simulink model "test01_Accumulator"  (Simulink 7.4)
settings: Solver=ode45  StartTime=0.0  StopTime=1.0  RelTol=1e-3
libraries: NAV420Lib x1
settings Model: Creator=djulzz  LastModifiedBy=djulzz

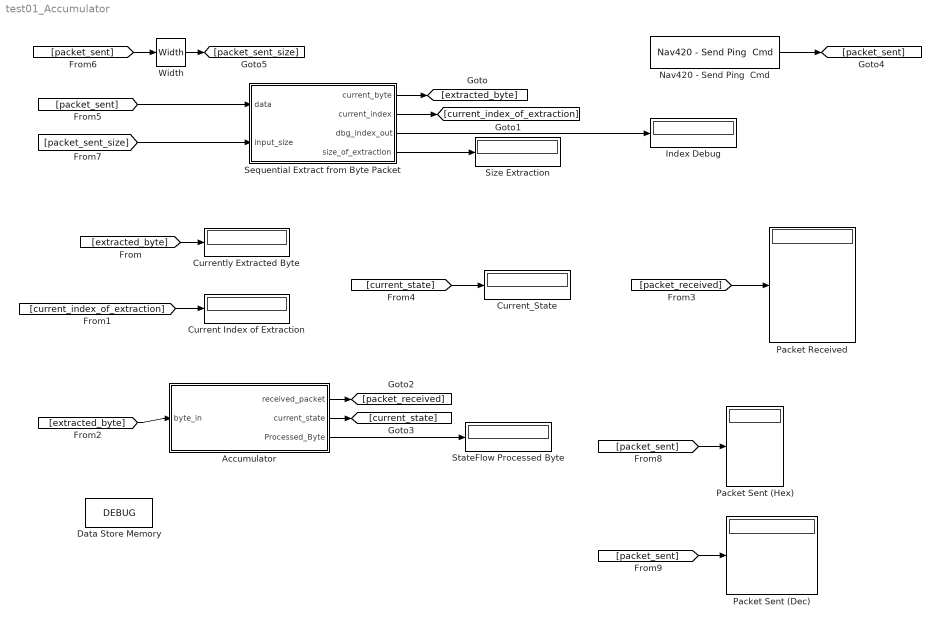
== system test01_Accumulator ==
  Accumulator : Subsystem
  Current Index of Extraction : Display
  Current_State : Display
  Currently Extracted Byte : Display
  Data Store Memory : DataStoreMemory  DataStoreName=DEBUG  DataType=double  OutDataType=fixdt(1, 16)  OutScaling=2^0  OutDataTypeStr=double
  Index Debug : Display
  Nav420 - Send Ping  Cmd : NAV420Lib/Nav420 - Send Ping  Cmd  SystemSampleTime=-1
  Packet Received : Display
  Packet Sent (Dec) : Display
  Packet Sent (Hex) : Display
      settings: Format=hex (Stored Integer)
  Sequential Extract from Byte Packet : Subsystem  TreatAsAtomicUnit=on
  Size Extraction : Display
  StateFlow Processed Byte : Display
      settings: Format=hex (Stored Integer)
  Width : Width
  wires:
  [extracted_byte] -> Currently Extracted Byte/1
  Sequential Extract from Byte Packet/1(current_byte) -> [extracted_byte]
  Sequential Extract from Byte Packet/2(current_index) -> [current_index_of_extraction]
  [current_index_of_extraction] -> Current Index of Extraction/1
  [extracted_byte] -> Accumulator/1(byte_in)
  Accumulator/1(received_packet) -> [packet_received]
  [packet_received] -> Packet Received/1
  [current_state] -> Current_State/1
  Accumulator/2(current_state) -> [current_state]
  Nav420 - Send Ping  Cmd/1 -> [packet_sent]
  [packet_sent] -> Sequential Extract from Byte Packet/1(data)
  [packet_sent] -> Width/1
  Width/1 -> [packet_sent_size]
  [packet_sent_size] -> Sequential Extract from Byte Packet/2(input_size)
  [packet_sent] -> Packet Sent (Hex)/1
  [packet_sent] -> Packet Sent (Dec)/1
  Accumulator/3(Processed_Byte) -> StateFlow Processed Byte/1
  Sequential Extract from Byte Packet/3(dbg_index_out) -> Index Debug/1
  Sequential Extract from Byte Packet/4(size_of_extraction) -> Size Extraction/1

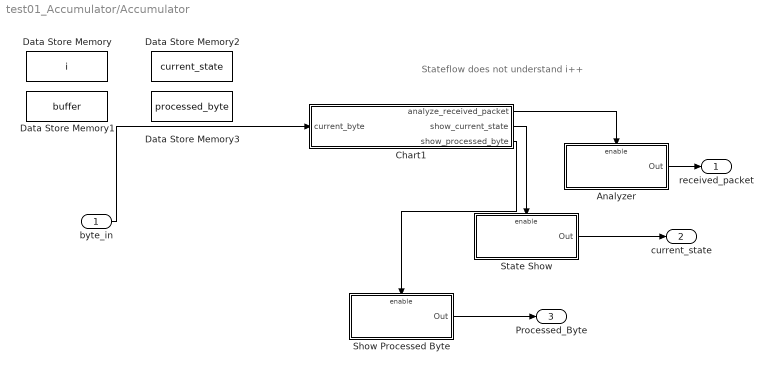
== system test01_Accumulator/Accumulator ==
  note: Stateflow does not understand i++
  byte_in : Inport  OutMin=[0]  OutMax=[255]  DataType=uint8  OutDataType=fixdt(1, 16)  OutScaling=2^0  OutDataTypeStr=uint8
  Analyzer : Subsystem  TreatAsAtomicUnit=on
  Chart1 : Stateflow chart
  Data Store Memory : DataStoreMemory  DataStoreName=i  InitialValue=1  OutMin=[0]  OutMax=[255]  DataType=uint8  OutDataType=fixdt(1, 16)  OutScaling=2^0  OutDataTypeStr=uint8
  Data Store Memory1 : DataStoreMemory  DataStoreName=buffer  InitialValue=[0 0 0 0 0 0 0 0 0 0 0 0 0 0 0 0 0 0 0 0 0 0 0 0 0 0 0 0 0 0 0 0 0 0 0 0 0 0 0 0 0 0 0 0 0 0 0 0 0 0 0 0 0 0 0 0 0 0 0 0 0 0 0 0 0 0 0 0 0 0 0 0 0 0 0 0 0 0 0 0 0 0 0 0 0 0 0 0 0 0 0 0 0 0 0 0 0 0 0 0]  DataType=uint8  OutDataType=fixdt(1, 16)  OutScaling=2^0  OutDataTypeStr=uint8
  Data Store Memory2 : DataStoreMemory  DataStoreName=current_state  DataType=double  OutDataType=fixdt(1, 16)  OutScaling=2^0  OutDataTypeStr=double
  Data Store Memory3 : DataStoreMemory  DataStoreName=processed_byte  DataType=uint8  OutDataType=fixdt(1, 16)  OutScaling=2^0  OutDataTypeStr=uint8
  Show Processed Byte : Subsystem  TreatAsAtomicUnit=on
  State Show : Subsystem  TreatAsAtomicUnit=on
  received_packet : Outport  DataType=uint8  OutDataType=fixdt(1, 16)  OutScaling=2^0  OutDataTypeStr=uint8
  current_state : Outport  Port=2  DataType=double  OutDataType=fixdt(1, 16)  OutScaling=2^0  OutDataTypeStr=double
  Processed_Byte : Outport  Port=3  DataType=uint8  OutDataType=fixdt(1, 16)  OutScaling=2^0  OutDataTypeStr=uint8
  wires:
  byte_in/1 -> Chart1/1(current_byte)
  Chart1/1(analyze_received_packet) -> Analyzer/Enable
  Analyzer/1(Out) -> received_packet/1
  Chart1/2(show_current_state) -> State Show/Enable
  State Show/1(Out) -> current_state/1
  Chart1/3(show_processed_byte) -> Show Processed Byte/Enable
  Show Processed Byte/1(Out) -> Processed_Byte/1

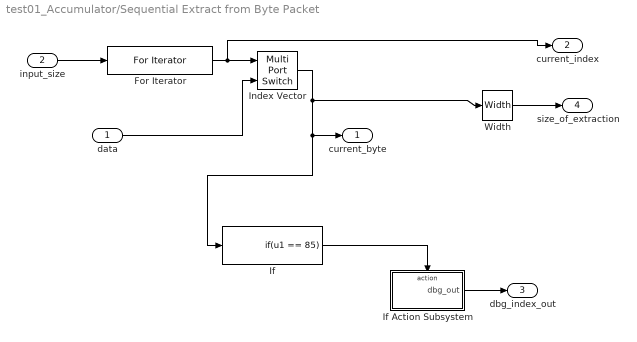
== system test01_Accumulator/Sequential Extract from Byte Packet ==
  data : Inport  OutDataType=fixdt(1, 16)  OutScaling=2^0
  input_size : Inport  Port=2  OutDataType=fixdt(1, 16)  OutScaling=2^0
  For Iterator : ForIterator  IterationSource=external
  If : If  IfExpression=u1 == 85  ShowElse=off
  If Action Subsystem : Subsystem  TreatAsAtomicUnit=on
  Index Vector : MultiPortSwitch  Inputs=1  OutDataTypeMode=uint8  OutDataType=fixdt(1, 16)  OutScaling=2^0  OutDataTypeStr=uint8
  Width : Width
  current_byte : Outport  DataType=uint8  OutDataType=fixdt(1, 16)  OutScaling=2^0  OutDataTypeStr=uint8
  current_index : Outport  Port=2  OutDataType=fixdt(1, 16)  OutScaling=2^0
  dbg_index_out : Outport  Port=3  DataType=double  OutDataType=fixdt(1, 16)  OutScaling=2^0  OutDataTypeStr=double
  size_of_extraction : Outport  Port=4  OutDataType=fixdt(1, 16)  OutScaling=2^0
  wires:
  input_size/1 -> For Iterator/1
  For Iterator/1 -> Index Vector/1, current_index/1
  data/1 -> Index Vector/2
  Index Vector/1 -> current_byte/1, If/1, Width/1
  If/1 -> If Action Subsystem/Action
  If Action Subsystem/1(dbg_out) -> dbg_index_out/1
  Width/1 -> size_of_extraction/1

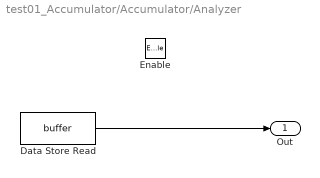
== system test01_Accumulator/Accumulator/Analyzer ==
  Enable : EnablePort  PropagateVarSize=During execution
  Data Store Read : DataStoreRead  DataStoreName=buffer  SampleTime=0
  Out : Outport  OutDataType=fixdt(1, 16)  OutScaling=2^0
  wires:
  Data Store Read/1 -> Out/1

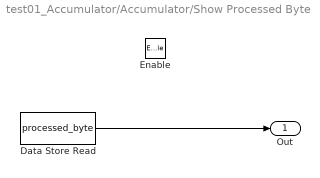
== system test01_Accumulator/Accumulator/Show Processed Byte ==
  Enable : EnablePort  PropagateVarSize=During execution
  Data Store Read : DataStoreRead  DataStoreName=processed_byte  SampleTime=0
  Out : Outport  DataType=uint8  OutDataType=fixdt(1, 16)  OutScaling=2^0  OutDataTypeStr=uint8
  wires:
  Data Store Read/1 -> Out/1

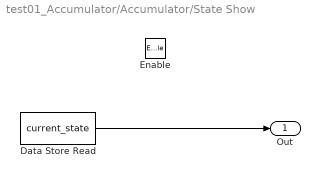
== system test01_Accumulator/Accumulator/State Show ==
  Enable : EnablePort  PropagateVarSize=During execution
  Data Store Read : DataStoreRead  DataStoreName=current_state  SampleTime=0
  Out : Outport  OutDataType=fixdt(1, 16)  OutScaling=2^0
  wires:
  Data Store Read/1 -> Out/1

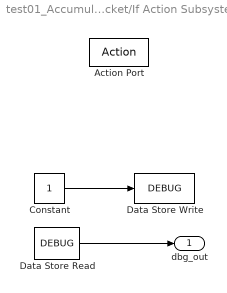
== system test01_Accumulator/Sequential Extract from Byte Packet/If Action Subsystem ==
  Action Port : ActionPort  ActionType=then
  Constant : Constant  OutDataTypeMode=double  OutDataType=fixdt(1, 16)  OutScaling=2^0  OutDataTypeStr=double
  Data Store Read : DataStoreRead  DataStoreName=DEBUG  SampleTime=-1
  Data Store Write : DataStoreWrite  DataStoreName=DEBUG  SampleTime=-1
  dbg_out : Outport  DataType=double  OutDataType=fixdt(1, 16)  OutScaling=2^0  OutDataTypeStr=double
  wires:
  Data Store Read/1 -> dbg_out/1
  Constant/1 -> Data Store Write/1

== stateflow chart Accumulator/Chart1 ==
  state First_Byte_of_Packet
    analyze_received_packet=1;
    current_state=1.0;
    show_current_state=1;
    processed_byte=current_byte;
    show_processed_byte=1;
    i=1;
  state First_U
    buffer[i]=current_byte;
    current_state=2.0;
    show_current_state=1;
    processed_byte=current_byte;
    show_processed_byte=1;
    i=i+1;
  state Bad_Start_Header
    current_state=-1.0;
    show_current_state=1;
    processed_byte=current_byte;
    show_processed_byte=1;
  (default) -> First_Byte_of_Packet
  First_Byte_of_Packet -> First_U [order 1] : [current_byte==85]
  First_Byte_of_Packet -> Bad_Start_Header [order 2] : [current_byte!=85]
  data: current_byte input uint8 size=1; buffer data_store_memory double; i data_store_memory double; analyze_received_packet output double; show_current_state output double; current_state data_store_memory double; processed_byte data_store_memory uint8; data local double; show_processed_byte output uint8
